simulink model "ACC_TEST_AEB_TEST_2011"  (Simulink 7.7)
settings: Solver=ode1  SolverMode=SingleTasking  StartTime=0.0  StopTime=T  FixedStep=0.001  RelTol=1e-3
PostLoadFcn:
  | , if any(exist('dsrtsu_mdlpostloadfcn', 'file') == [2, 3, 6]), try dsrtsu_mdlpostloadfcn('Execute', bdroot); catch fprintf('Error in PostLoadFcn (dsrtsu_mdlpostloadfcn) for model "%s":\n %s\n', bdroot, lasterr); end, end,
model workspace (MATLAB code in the model file):
  | % Define the sample time, |Ts|, and simulation duration, |T|, in seconds.
  | Ts = 0.1;
  | T = 35;
  | 
  | % Specify the initial position and velocity for the two vehicles.
  | % v0_lead_long = 20;
  | v0_lead_long = 15;
  | v0_lead_lat = 1;  % initial velocity for lead car (m/s)
  | x0_target = 45.15;            % Initial x position of target car          (m)
  | y0_target = 1.933;       % Initial y position of target car          (m)
  | % x0_target = 0;            % Initial x position of target car          (m)
  | % y0_target = 0;       % Initial y position of target car          (m)
  | lead_heading = 0.09;
  | yaw_des = 0.09;
  | 
  | % Initial condition for the ego car
  | x0_egoVehicle = [0 0];   % initial position for ego car (m)
  | v0_ego = 20;   % initial velocity for ego car (m/s)
  | % Initial condition for the ego car
  | % v0_ego = 20.6;         % Initial speed of the ego car           (m/s)
  | x0_ego = 0;            % Initial x position of ego car          (m)
  | y0_ego = 0;       % Initial y position of ego car          (m)
  | 
  | t_gap = 1.4;
  | D_default = 10;
  | %%
  | % Specify the driver-set velocity in m/s.
  | % v_set = 30;
  | 
  | %%
  | % Considering the physical limitations of the vehicle dynamics, the
  | % acceleration is constrained to the range  |[-3,2]| (m/s^2).
  | min_ac = -3;
  | max_ac = 2;
  | max_jerk = 90;
  | min_jerk =-90;
  | R           = 500;      % Radius of curvature for the road      (m)
  | %% Ego Car
  | % Dynamics modeling parameters
  | m       = 1575;     % Total mass of vehicle                          (kg)
  | Iz      = 2875;     % Yaw moment of inertia of vehicle               (m*N*s^2)
  | lf      = 1.2;      % Longitudinal distance from c.g. to front tires (m)
  | lr      = 1.6;      % Longitudinal distance from c.g. to rear tires  (m)
  | Cf      = 19000;    % Cornering stiffness of front tires             (N/rad)
  | Cr      = 33000;    % Cornering stiffness of rear tires              (N/rad)
  | tau     = 0.5;      % Longitudinal time constant                     (N/A)
  | 
  | % System matrices
  | A = [-(2*Cf+2*Cr)/m/v0_ego,0,-v0_ego-(2*Cf*lf-2*Cr*lr)/m/v0_ego,0,0;...
  |      0,0,1,0,0;...
  |      -(2*Cf*lf-2*Cr*lr)/Iz/v0_ego,0,-(2*Cf*lf^2+2*Cr*lr^2)/Iz/v0_ego,0,0;...
  |      0,0,0,0,1;...
  |      0,0,0,0,-1/tau];
  | % B1 = [2*Cf/m,0,2*Cf*lf/Iz,0,0]';
  | B2 = [0,0,0,0,1/tau]';
  | 
  | %% Linear Model for ACC design
  | % Input:  u (required longitudinal acceleration)
  | % Output: x4(longitudinal velocity)
  | C = [0,0,0,1,0];
  | G = minreal(ss(A,B2,C,0));
  | 
  | %% Driver steering control paramaters
  | driver_P        = 0.2;  % Proportional gain                     (N/A)
  | driver_I        = 0.1;  % Integral gain                         (N/A)
  | yawerr_gain     = 2;    % Yaw error gain                        (N/A)
  | 
  | %% Automatic Cruise Control (ACC) Controller Parameters
  | v_set           = 20; % ACC set speed                         (m/s)
  | time_gap        = 1;  % ACC time gap                          (s)
  | default_spacing = 5;    % ACC default spacing                   (m)
  | verr_gain       = 5;  % ACC velocity error gain               (N/A)
  | xerr_gain       = 0.2;  % ACC spacing error gain                (N/A)
  | vx_gain         = 0.1;  % ACC relative velocity gain            (N/A)
  | 
  | %% AEB
  | tau1     = 0.5;     % Longitudinal time constant (throttle)          (N/A)
  | tau2     = 0.07;    % Longitudinal time constant (brake)             (N/A)
  | v_set_aeb = 20;
  | 
  | %% Speed Controller Parameters
  | speedController.Kp = 1.1;           % Proportional Gain of speed controller
  | speedController.Ki = 0.1;           % Integral Gain of speed controller
  | speedController.Amax = 3;           % Maximum acceleration                  (m/s^2)
  | speedController.Amin = -3;          % Minimum acceleration                  (m/s^2)
  | 
  | %% FCW parameters
  | FCW.timeToReact  = 1.2;         % driver reaction time                   (sec)
  | FCW.driver_decel = 4.0;         % driver braking deceleration            (m/s^2)
  | 
  | %% AEB controller parameters
  | AEB.PB1_decel = 3.8;            % 1st stage Partial Braking deceleration (m/s^2)
  | AEB.PB2_decel = 5.3;            % 2nd stage Partial Braking deceleration (m/s^2)
  | AEB.FB_decel  = 9.8;            % Full Braking deceleration              (m/s^2)
  | AEB.headwayOffset = 3.7;        % headway offset                         (m)
  | AEB.timeMargin = 0;             % headway time margin                    (sec)
libraries: simulink x4
Description:
  | Standard RTI1401 template.
  | Supported Matlab version:  R2017a.
settings Model: Tag=RTI1401  DSRTSU_INTERNAL_RTI_VER=510  DSRTSU_INTERNAL_RTI_TYPE=rti1401  RTICANMMDATA=struct('GeneralSetupData',struct('modelroot',['C:\Users\pegas\Desktop\MDS\Desktop\Matlab Ex'],'generalsettings',struct('filesettings',struct('destfolder',struct('Name','RTICANMM_FILES','Check',1),'buildfolder',struct('Name','.','Check',1),'AbsDestfolder',struct('Name',['C:\Users\pegas\Desktop\MDS\Desktop\Matlab Ex\RTICANMM_FILES']),'AbsBuildfolder',struct('Name',['C:\Users\pegas\Desktop\MDS\Desktop\Matlab Ex']))),'options',struct('addpaths',1,'rmpaths',1,'addtrcexclusion',logical(1),'cannavigator',struct('checkmonitoring',0),'show_usrtrc',0,'use_usrtrc',0),'advanced',struct('options',[1 1 1 1 1 1 1 1 1 1 1 1 1 1 1 1 1 1 1 1 1 1 1 1 1 1 1 1 1 1 1 1 1 1 1 1 1 1 1 1 1 1 1 1 1 1 1 1 1 1 1 1 1 1 1 1 1 1 1 1 1 1 1 1 1 1 1 1 1 1 1 1 1 1 1 1 1 1 1 1 1 1 1 1 1 1 1 1 1 1 1 1 1 1 1 1 1 1 1 1]),'MPSetup',{{}},'modelname','ACC_TEST_AEB_TEST_2017','block','ACC_TEST_AEB_TEST_2017'))  DSRTSU_INTERNAL_RTIFLEXRAYCONFIG=110  DSRTSU_INTERNAL_RTIFPGA=110  Creator=pegas  LastModifiedBy=pegas  CovMetricSettings=dswe  CovHtmlReporting=off  covSaveCumulativeToWorkspaceVar=off  CovSaveSingleToWorkspaceVar=off  CovExternalEMLEnable=on
settings DataIOCC: LimitDataPoints=off  SaveFormat=StructureWithTime  SignalLoggingSaveFormat=Dataset
settings OptimizationCC: BlockReduction=off  OptimizeBlockIOStorage=off  BufferReuse=off  ExpressionFolding=off  ExpressionDepthLimit=128  LocalBlockOutputs=off
settings DebuggingCC: UnderspecifiedInitializationDetection=Simplified  MergeDetectMultiDrivingBlocksExec=error  SolverPrmCheckMsg=none  FcnCallInpInsideContextMsg=Enable All  StateNameClashWarn=none  SFUnexpectedBacktrackingDiag=error  SFNoUnconditionalDefaultTransitionDiag=error
settings HardwareCC: ProdLargestAtomicInteger=Integer  ProdLargestAtomicFloat=Float  ProdIntDivRoundTo=Zero  ProdEndianess=BigEndian  ProdHWDeviceType=Custom Processor->Custom  TargetIntDivRoundTo=Zero  TargetEndianess=BigEndian  TargetHWDeviceType=Custom Processor->Custom
settings RTWCC: SystemTargetFile=rti1401.tlc  MakeCommand=make_rti  TemplateMakefile=rti1401.tmf  Description=dSPACE DS1401 Hardware Platform
settings CodeAppCC: CustomSymbolStrType=$N$R$M_T
settings STFCustomTargetCC: TargetFunctionLibrary=C89/C90 (ANSI)  ParMdlRefBuildCompliant=on  MatFileLogging=on  SystemTargetFile=rti1401.tlc
settings GRTTargetCC: TargetFunctionLibrary=C89/C90 (ANSI)  CompOptLevelCompliant=off  GeneratePreprocessorConditionals=Use local settings
settings CustomProperty: DataType=RTWOptions_EnumType_C__Program Files_dSPACE RCPHIL 2017-B_MATLAB_RTI_RTI1401_TLC_rti1401_1InitialSimState  Value=RUN
settings EnumStrPairs: String=RUN

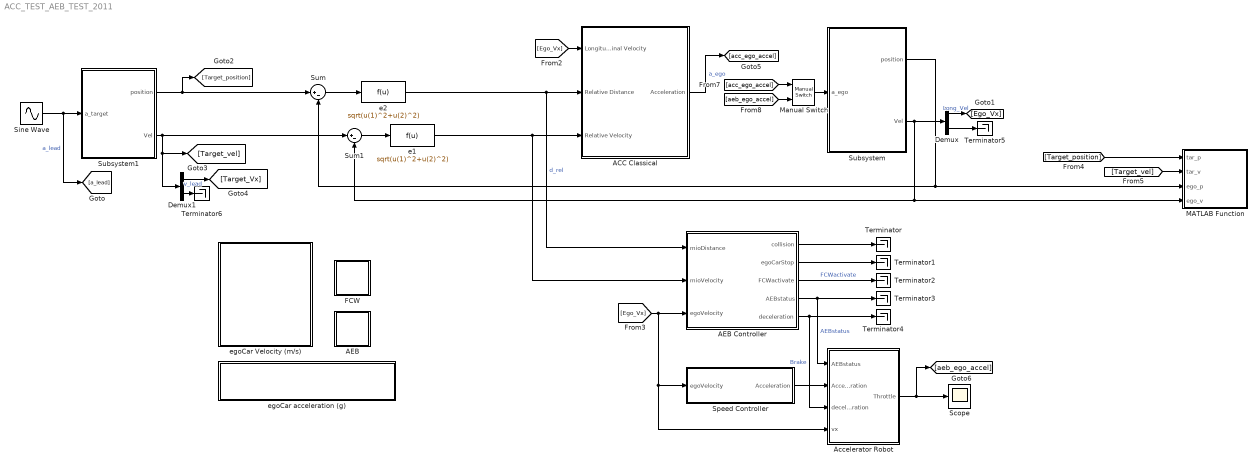
== system ACC_TEST_AEB_TEST_2011 ==
  ACC Classical : Subsystem  TreatAsAtomicUnit=on  VariantObject=controller_type == 1
      settings: RTWFileNameOpts=Use function name
  AEB : Subsystem  Description=Replaced Block
      mask Type: Replaced Block
      mask Description: This block has been replaced with an empty subsystem because it used functionality that is unavailable in Simulink R2011a.
      mask Display: fprintf('Replaced: %s\n','Dashboard Widget')
  AEB Controller : Subsystem
  Accelerator Robot : Subsystem
  Demux : Demux  Outputs=2
  Demux1 : Demux  Outputs=2
  FCW : Subsystem  Description=Replaced Block
      mask Type: Replaced Block
      mask Description: This block has been replaced with an empty subsystem because it used functionality that is unavailable in Simulink R2011a.
      mask Display: fprintf('Replaced: %s\n','Dashboard Widget')
  MATLAB Function : Stateflow chart  TreatAsAtomicUnit=on
      settings: PermitHierarchicalResolution=ParametersOnly
  Manual Switch : simulink/Signal Routing/Manual Switch  sw=1  action=0  varsize=off
  Scope : Scope
      settings: TimeRange=auto  MaxDataPoints=5000  SaveToWorkspace=off  YMin=-1.25  YMax=1.25  SampleTime=-1
  Sine Wave : Sin  Amplitude=0.6  Frequency=0.2  SampleTime=Ts
  Speed Controller : Subsystem
  Subsystem : Subsystem
  Subsystem1 : Subsystem
  Sum : Sum  Inputs=|+-
  Sum1 : Sum  Inputs=|+-
  Terminator{,1..6} (7 alike) : Terminator
  e1 : Fcn  Expr=sqrt(u(1)^2+u(2)^2)
  e2 : Fcn  Expr=sqrt(u(1)^2+u(2)^2)
  egoCar Velocity (m/s) : Subsystem  Description=Replaced Block
      mask Type: Replaced Block
      mask Description: This block has been replaced with an empty subsystem because it used functionality that is unavailable in Simulink R2011a.
      mask Display: fprintf('Replaced: %s\n','Dashboard Widget')
  egoCar acceleration (g) : Subsystem  Description=Replaced Block
      mask Type: Replaced Block
      mask Description: This block has been replaced with an empty subsystem because it used functionality that is unavailable in Simulink R2011a.
      mask Display: fprintf('Replaced: %s\n','Dashboard Widget')
  wires:
  Sum1/1 -> e1/1
  Sum/1 -> e2/1
  Subsystem1/1(position) -> [Target_position], Sum/1
  Subsystem1/2(Vel) -> Sum1/1, [Target_vel], Demux1/1
  Subsystem/2(Vel) -> Sum1/2, MATLAB Function/4(ego_v), Demux/1
  e1/1 -> ACC Classical/3(Relative Velocity), AEB Controller/2(mioVelocity)
  Subsystem/1(position) -> Sum/2, MATLAB Function/3(ego_p)
  Sine Wave/1 -> [a_lead], Subsystem1/1(a_target)  "a_lead"
  e2/1 -> ACC Classical/2(Relative Distance), AEB Controller/1(mioDistance)  "d_rel"
  AEB Controller/1(collision) -> Terminator/1
  AEB Controller/2(egoCarStop) -> Terminator1/1
  AEB Controller/3(FCWactivate) -> Terminator2/1  "FCWactivate"
  AEB Controller/4(AEBstatus) -> Terminator3/1, Accelerator Robot/1(AEBstatus)  "AEBstatus"
  AEB Controller/5(deceleration) -> Terminator4/1, Accelerator Robot/3(decelleration)  "Brake"
  Demux/2 -> Terminator5/1
  Demux/1 -> [Ego_Vx]  "Long_Vel"
  Speed Controller/1(Acceleration) -> Accelerator Robot/2(Acceleration)
  Accelerator Robot/1(Throttle) -> [aeb_ego_accel], Scope/1
  ACC Classical/1(Acceleration) -> [acc_ego_accel]  "a_ego"
  [Ego_Vx] -> ACC Classical/1(Longitudinal Velocity)
  [Ego_Vx] -> AEB Controller/3(egoVelocity), Accelerator Robot/4(vx), Speed Controller/1(egoVelocity)
  [Target_position] -> MATLAB Function/1(tar_p)
  [Target_vel] -> MATLAB Function/2(tar_v)
  Demux1/2 -> Terminator6/1
  Demux1/1 -> [Target_Vx]  "v_lead"
  Manual Switch/1 -> Subsystem/1(a_ego)
  [acc_ego_accel] -> Manual Switch/1
  [aeb_ego_accel] -> Manual Switch/2

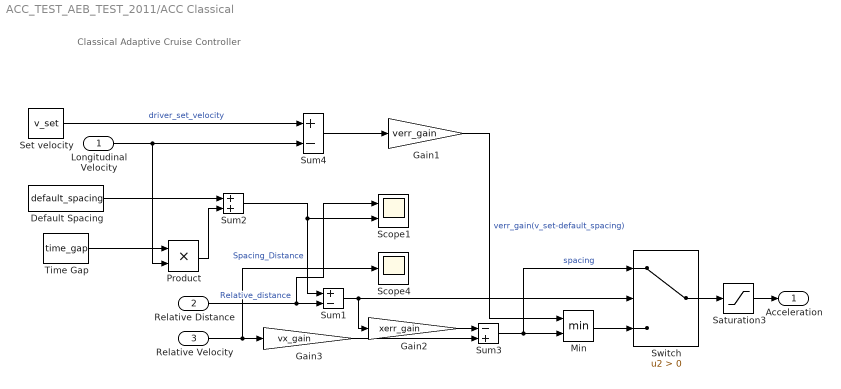
== system ACC_TEST_AEB_TEST_2011/ACC Classical ==
  note: Classical Adaptive Cruise Controller
  Longitudinal Velocity : Inport
  Relative Distance : Inport  Port=2
  Relative Velocity : Inport  Port=3
  Default Spacing : Constant  Value=default_spacing  SampleTime=Ts
  Gain1 : Gain  Gain=verr_gain
  Gain2 : Gain  Gain=xerr_gain
  Gain3 : Gain  Gain=vx_gain
  Min : MinMax  Inputs=2
  Product : Product
  Saturation3 : Saturate  UpperLimit=max_ac  LowerLimit=min_ac
  Scope1 : Scope  NumInputPorts=2
      settings: TimeRange=auto  MaxDataPoints=5000  SaveToWorkspace=off  YMin=-3.97675~-5  YMax=50.65448~5  SampleTime=-1
  Scope4 : Scope
      settings: TimeRange=auto  MaxDataPoints=5000  SaveToWorkspace=off  SaveName=ScopeData6  YMin=-0.54934  YMax=6.34874  SampleTime=-1
  Set velocity : Constant  Value=v_set  SampleTime=Ts
  Sum1 : Sum  Inputs=+-
  Sum2 : Sum
  Sum3 : Sum  Inputs=-+
  Sum4 : Sum  Inputs=+-
  Switch : Switch  Criteria=u2 > Threshold
  Time Gap : Constant  Value=time_gap  SampleTime=Ts
  Acceleration : Outport
  wires:
  Longitudinal Velocity/1 -> Product/2, Sum4/2
  Default Spacing/1 -> Sum2/1
  Gain2/1 -> Sum3/1
  Sum4/1 -> Gain1/1
  Gain3/1 -> Sum3/2
  Relative Velocity/1 -> Scope4/1, Gain3/1
  Time Gap/1 -> Product/1
  Switch/1 -> Saturation3/1
  Product/1 -> Sum2/2
  Set velocity/1 -> Sum4/1  "driver_set_velocity"
  Sum3/1 -> Switch/1, Min/2  "spacing"
  Sum1/1 -> Gain2/1, Switch/2
  Gain1/1 -> Min/1  "verr_gain(v_set-default_spacing)"
  Relative Distance/1 -> Scope1/1, Sum1/2  "Relative_distance"
  Sum2/1 -> Scope1/2, Sum1/1  "Spacing_Distance"
  Saturation3/1 -> Acceleration/1
  Min/1 -> Switch/3

== system ACC_TEST_AEB_TEST_2011/AEB ==

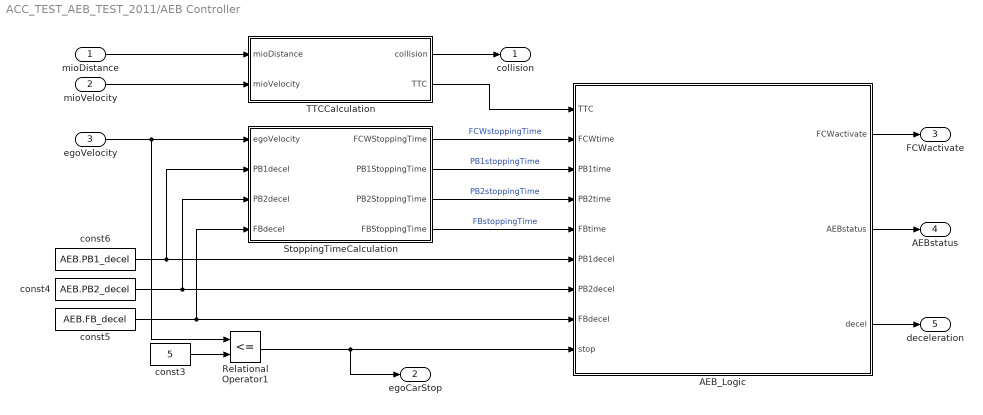
== system ACC_TEST_AEB_TEST_2011/AEB Controller ==
  mioDistance : Inport
  mioVelocity : Inport  Port=2
  egoVelocity : Inport  Port=3
  AEB_Logic : Stateflow chart  TreatAsAtomicUnit=on
      settings: PermitHierarchicalResolution=ParametersOnly
  Relational Operator1 : RelationalOperator  Operator=<=  OutDataTypeStr=boolean
  StoppingTimeCalculation : Subsystem
  TTCCalculation : Subsystem
  const3 : Constant  Value=5  SampleTime=-1
  const4 : Constant  Value=AEB.PB2_decel  SampleTime=-1
  const5 : Constant  Value=AEB.FB_decel  SampleTime=-1
  const6 : Constant  Value=AEB.PB1_decel  SampleTime=-1
  collision : Outport
  egoCarStop : Outport  Port=2
  FCWactivate : Outport  Port=3
  AEBstatus : Outport  Port=4
  deceleration : Outport  Port=5
  wires:
  AEB_Logic/3(decel) -> deceleration/1
  egoVelocity/1 -> StoppingTimeCalculation/1(egoVelocity), Relational Operator1/1
  const4/1 -> AEB_Logic/7(PB2decel), StoppingTimeCalculation/3(PB2decel)
  const5/1 -> StoppingTimeCalculation/4(FBdecel), AEB_Logic/8(FBdecel)
  AEB_Logic/2(AEBstatus) -> AEBstatus/1
  const3/1 -> Relational Operator1/2
  Relational Operator1/1 -> egoCarStop/1, AEB_Logic/9(stop)
  const6/1 -> AEB_Logic/6(PB1decel), StoppingTimeCalculation/2(PB1decel)
  StoppingTimeCalculation/3(PB2StoppingTime) -> AEB_Logic/4(PB2time)  "PB2stoppingTime"
  StoppingTimeCalculation/2(PB1StoppingTime) -> AEB_Logic/3(PB1time)  "PB1stoppingTime"
  StoppingTimeCalculation/4(FBStoppingTime) -> AEB_Logic/5(FBtime)  "FBstoppingTime"
  StoppingTimeCalculation/1(FCWStoppingTime) -> AEB_Logic/2(FCWtime)  "FCWstoppingTime"
  AEB_Logic/1(FCWactivate) -> FCWactivate/1
  mioDistance/1 -> TTCCalculation/1(mioDistance)
  mioVelocity/1 -> TTCCalculation/2(mioVelocity)
  TTCCalculation/1(collision) -> collision/1
  TTCCalculation/2(TTC) -> AEB_Logic/1(TTC)

== system ACC_TEST_AEB_TEST_2011/Accelerator Robot ==
  note: Robot release accelerator when AEB is activated
  AEBstatus : Inport
  Acceleration : Inport  Port=2
  decelleration : Inport  Port=3
  vx : Inport  Port=4
  Constant : Constant  Value=0
  Saturation : Saturate  UpperLimit=1  LowerLimit=-1
  Simple Driveline & Brakes : Subsystem
  Switch : Switch  Criteria=u2 > Threshold
  Throttle : Outport
  wires:
  Constant/1 -> Switch/1
  decelleration/1 -> Simple Driveline & Brakes/2(Brake)
  Switch/1 -> Simple Driveline & Brakes/1(Throttle)
  Simple Driveline & Brakes/1(Accel) -> Saturation/1
  Acceleration/1 -> Switch/3
  vx/1 -> Simple Driveline & Brakes/3(xdot)
  Saturation/1 -> Throttle/1
  AEBstatus/1 -> Switch/2

== system ACC_TEST_AEB_TEST_2011/FCW ==

== system ACC_TEST_AEB_TEST_2011/Speed Controller ==
  egoVelocity : Inport
  Discrete PID Controller2 : simulink/Continuous/PID Controller  Controller=PI  TimeDomain=Discrete-time  SampleTime=-1  IntegratorMethod=Forward Euler  FilterMethod=Forward Euler  Form=Parallel  UseFilter=on  ControllerParametersSource=internal  P=speedController.Kp  I=speedController.Ki  D=speedController.Kd  N=speedController.FilterCoeff  InitialConditionSource=internal  InitialConditionForIntegrator=0  InitialConditionForFilter=0  ExternalReset=none  LimitOutput=on  UpperSaturationLimit=speedController.Amax  LowerSaturationLimit=speedController.Amin  LinearizeAsGain=off  AntiWindupMode=clamping  Kb=1  TrackingMode=off  Kt=1  PParamMin=[]  PParamMax=[]  IParamMin=[]  IParamMax=[]  DParamMin=[]  DParamMax=[]  NParamMin=[]  NParamMax=[]  KbParamMin=[]  KbParamMax=[]  KtParamMin=[]  KtParamMax=[]  POutMin=[]  POutMax=[]  IOutMin=[]  IOutMax=[]  DOutMin=[]  DOutMax=[]  NOutMin=[]  NOutMax=[]  KbOutMin=[]  KbOutMax=[]  KtOutMin=[]  KtOutMax=[]  IntegratorOutMin=[]  IntegratorOutMax=[]  FilterOutMin=[]  FilterOutMax=[]  SumOutMin=[]  SumOutMax=[]  SumI1OutMin=[]  SumI1OutMax=[]  SumI2OutMin=[]  SumI2OutMax=[]  SumI3OutMin=[]  SumI3OutMax=[]  SumDOutMin=[]  SumDOutMax=[]  SaturationOutMin=[]  SaturationOutMax=[]  IntegratorContinuousStateAttributes=''  IntegratorStateMustResolveToSignalObject=off  IntegratorRTWStateStorageClass=Auto  FilterContinuousStateAttributes=''  FilterStateMustResolveToSignalObject=off  FilterRTWStateStorageClass=Auto  DifferentiatorICPrevScaledInput=0  DifferentiatorOutMin=[]  DifferentiatorOutMax=[]
  Set velocity : Constant  Value=v_set_aeb  SampleTime=Ts
  Sum4 : Sum  Inputs=+-
  Acceleration : Outport
  wires:
  Set velocity/1 -> Sum4/1  "driver_set_velocity"
  egoVelocity/1 -> Sum4/2
  Discrete PID Controller2/1 -> Acceleration/1
  Sum4/1 -> Discrete PID Controller2/1

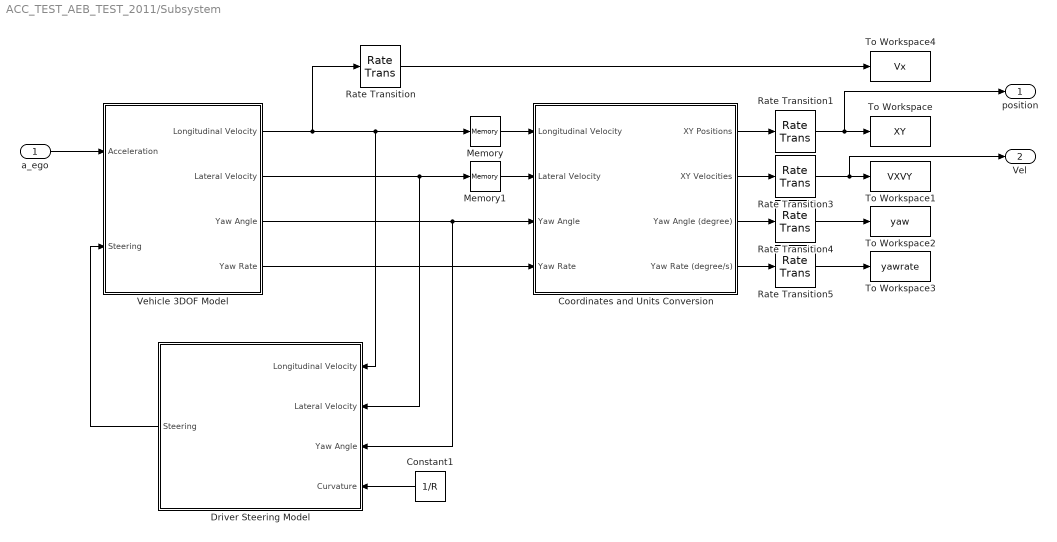
== system ACC_TEST_AEB_TEST_2011/Subsystem ==
  a_ego : Inport
  "  Vehicle 3DOF Model " : Subsystem
  Constant1 : Constant  Value=1/R
  Coordinates and Units Conversion : Subsystem
  Driver Steering Model : Subsystem
  Memory : Memory  X0=v0_ego
  Memory1 : Memory
  Rate Transition{,1,3..5} (5 alike) : RateTransition  OutPortSampleTime=Ts
  To Workspace : ToWorkspace  VariableName=XY  SaveFormat=Structure With Time  SampleTime=-1
  To Workspace1 : ToWorkspace  VariableName=VXVY  SaveFormat=Structure With Time  SampleTime=-1
  To Workspace2 : ToWorkspace  VariableName=yaw  SaveFormat=Structure With Time  SampleTime=-1
  To Workspace3 : ToWorkspace  VariableName=yawrate  SaveFormat=Structure With Time  SampleTime=-1
  To Workspace4 : ToWorkspace  VariableName=Vx  SaveFormat=Structure With Time  SampleTime=-1
  position : Outport
  Vel : Outport  Port=2
  wires:
  Coordinates and Units Conversion/3(Yaw Angle (degree)) -> Rate Transition4/1
  Rate Transition5/1 -> To Workspace3/1
  "  Vehicle 3DOF Model "/2(Lateral Velocity) -> Memory1/1, Driver Steering Model/2(Lateral Velocity)
  Rate Transition/1 -> To Workspace4/1
  Constant1/1 -> Driver Steering Model/4(Curvature)
  Coordinates and Units Conversion/1(XY Positions) -> Rate Transition1/1
  "  Vehicle 3DOF Model "/1(Longitudinal Velocity) -> Rate Transition/1, Driver Steering Model/1(Longitudinal Velocity), Memory/1
  Driver Steering Model/1(Steering) -> "  Vehicle 3DOF Model "/2(Steering)
  Rate Transition4/1 -> To Workspace2/1
  "  Vehicle 3DOF Model "/3(Yaw Angle) -> Coordinates and Units Conversion/3(Yaw Angle), Driver Steering Model/3(Yaw Angle)
  Coordinates and Units Conversion/4(Yaw Rate (degree/s)) -> Rate Transition5/1
  "  Vehicle 3DOF Model "/4(Yaw Rate) -> Coordinates and Units Conversion/4(Yaw Rate)
  Coordinates and Units Conversion/2(XY Velocities) -> Rate Transition3/1
  a_ego/1 -> "  Vehicle 3DOF Model "/1(Acceleration)
  Rate Transition1/1 -> position/1, To Workspace/1
  Rate Transition3/1 -> Vel/1, To Workspace1/1
  Memory/1 -> Coordinates and Units Conversion/1(Longitudinal Velocity)
  Memory1/1 -> Coordinates and Units Conversion/2(Lateral Velocity)

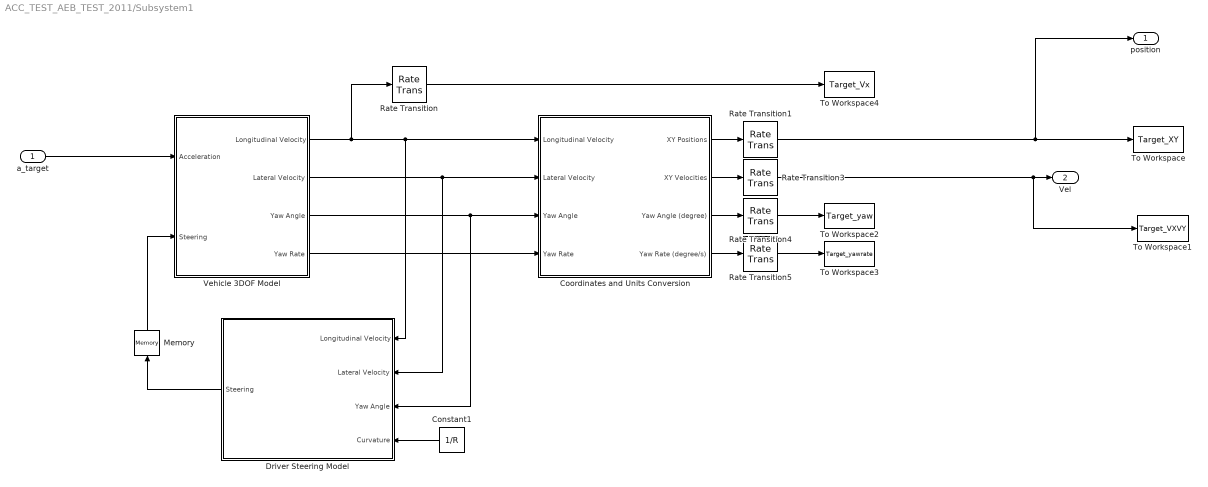
== system ACC_TEST_AEB_TEST_2011/Subsystem1 ==
  a_target : Inport
  "  Vehicle 3DOF Model " : Subsystem
  Constant1 : Constant  Value=1/R
  Coordinates and Units Conversion : Subsystem
  Driver Steering Model : Subsystem
  Memory : Memory  X0=0.01
  Rate Transition{,1,3..5} (5 alike) : RateTransition  OutPortSampleTime=Ts
  To Workspace : ToWorkspace  VariableName=Target_XY  SaveFormat=Structure With Time  SampleTime=-1
  To Workspace1 : ToWorkspace  VariableName=Target_VXVY  SaveFormat=Structure With Time  SampleTime=-1
  To Workspace2 : ToWorkspace  VariableName=Target_yaw  SaveFormat=Structure With Time  SampleTime=-1
  To Workspace3 : ToWorkspace  VariableName=Target_yawrate  SaveFormat=Structure With Time  SampleTime=-1
  To Workspace4 : ToWorkspace  VariableName=Target_Vx  SaveFormat=Structure With Time  SampleTime=-1
  position : Outport
  Vel : Outport  Port=2
  wires:
  a_target/1 -> "  Vehicle 3DOF Model "/1(Acceleration)
  Coordinates and Units Conversion/2(XY Velocities) -> Rate Transition3/1
  "  Vehicle 3DOF Model "/4(Yaw Rate) -> Coordinates and Units Conversion/4(Yaw Rate)
  Coordinates and Units Conversion/4(Yaw Rate (degree/s)) -> Rate Transition5/1
  "  Vehicle 3DOF Model "/3(Yaw Angle) -> Driver Steering Model/3(Yaw Angle), Coordinates and Units Conversion/3(Yaw Angle)
  Rate Transition4/1 -> To Workspace2/1
  Coordinates and Units Conversion/1(XY Positions) -> Rate Transition1/1
  Constant1/1 -> Driver Steering Model/4(Curvature)
  Rate Transition/1 -> To Workspace4/1
  Rate Transition5/1 -> To Workspace3/1
  Coordinates and Units Conversion/3(Yaw Angle (degree)) -> Rate Transition4/1
  Rate Transition1/1 -> position/1, To Workspace/1
  Rate Transition3/1 -> To Workspace1/1, Vel/1
  "  Vehicle 3DOF Model "/1(Longitudinal Velocity) -> Coordinates and Units Conversion/1(Longitudinal Velocity), Driver Steering Model/1(Longitudinal Velocity), Rate Transition/1
  "  Vehicle 3DOF Model "/2(Lateral Velocity) -> Coordinates and Units Conversion/2(Lateral Velocity), Driver Steering Model/2(Lateral Velocity)
  Driver Steering Model/1(Steering) -> Memory/1
  Memory/1 -> "  Vehicle 3DOF Model "/2(Steering)

== system ACC_TEST_AEB_TEST_2011/egoCar Velocity (m/s) ==

== system ACC_TEST_AEB_TEST_2011/egoCar acceleration (g) ==

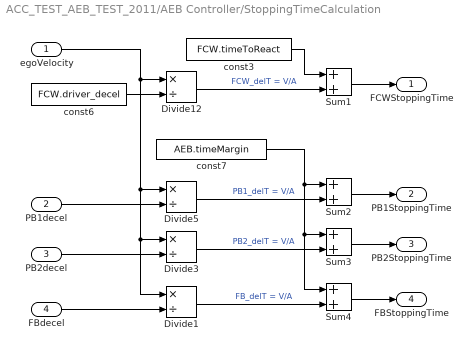
== system ACC_TEST_AEB_TEST_2011/AEB Controller/StoppingTimeCalculation ==
  egoVelocity : Inport
  PB1decel : Inport  Port=2
  PB2decel : Inport  Port=3
  FBdecel : Inport  Port=4
  Divide{1,3,5,12} (4 alike) : Product  Inputs=*/
  Sum{1..4} (4 alike) : Sum
  const3 : Constant  Value=FCW.timeToReact  SampleTime=-1
  const6 : Constant  Value=FCW.driver_decel  SampleTime=-1
  const7 : Constant  Value=AEB.timeMargin  SampleTime=-1
  FCWStoppingTime : Outport
  PB1StoppingTime : Outport  Port=2
  PB2StoppingTime : Outport  Port=3
  FBStoppingTime : Outport  Port=4
  wires:
  Sum1/1 -> FCWStoppingTime/1
  Sum2/1 -> PB1StoppingTime/1
  Sum3/1 -> PB2StoppingTime/1
  Sum4/1 -> FBStoppingTime/1
  const7/1 -> Sum2/1, Sum4/1, Sum3/1
  egoVelocity/1 -> Divide1/1, Divide3/1, Divide5/1, Divide12/1
  Divide5/1 -> Sum2/2  "PB1_delT = V/A"
  Divide3/1 -> Sum3/2  "PB2_delT = V/A"
  Divide1/1 -> Sum4/2  "FB_delT = V/A"
  const6/1 -> Divide12/2
  PB1decel/1 -> Divide5/2
  PB2decel/1 -> Divide3/2
  FBdecel/1 -> Divide1/2
  const3/1 -> Sum1/1
  Divide12/1 -> Sum1/2  "FCW_delT = V/A"

== system ACC_TEST_AEB_TEST_2011/AEB Controller/TTCCalculation ==
  mioDistance : Inport
  mioVelocity : Inport  Port=2
  Abs : Abs
  Divide11 : Product  Inputs=**
  Divide3 : Product  Inputs=*/
  Relational Operator : RelationalOperator  Operator=<  OutDataTypeStr=boolean
  Saturation : Saturate  UpperLimit=100  LowerLimit=0.01
  Sign : Signum
  Sum : Sum  Inputs=+-
  const1 : Constant  Value=AEB.headwayOffset  SampleTime=-1
  const2 : Constant  Value=0.1  SampleTime=-1
  collision : Outport
  TTC : Outport  Port=2
  wires:
  mioVelocity/1 -> Sign/1, Abs/1
  mioDistance/1 -> Sum/1
  Divide3/1 -> Divide11/1  "TTC"
  const1/1 -> Sum/2
  Sum/1 -> Relational Operator/1, Divide3/1  "headway"
  const2/1 -> Relational Operator/2
  Abs/1 -> Saturation/1
  Relational Operator/1 -> collision/1
  Saturation/1 -> Divide3/2
  Sign/1 -> Divide11/2
  Divide11/1 -> TTC/1  "TTC"

== system ACC_TEST_AEB_TEST_2011/Accelerator Robot/Simple Driveline & Brakes ==
  Throttle : Inport
  Brake : Inport  Port=2
  xdot : Inport  Port=3
  Gain : Gain  Gain=m
  Gain1 : Gain  Gain=0.8
  Gain2 : Gain  Gain=m
  Lower level dynamics1 : TransferFcn  Denominator=[tau1 1]
  Lower level dynamics2 : TransferFcn  Denominator=[tau2 1]
  Product : Product
  Subtract1 : Sum  Inputs=+-
  Trigonometric Function : Trigonometry  Operator=tanh
  Accel : Outport
  wires:
  Brake/1 -> Product/1
  Throttle/1 -> Gain/1
  Gain2/1 -> Lower level dynamics2/1
  Gain/1 -> Lower level dynamics1/1
  Subtract1/1 -> Accel/1
  xdot/1 -> Gain1/1
  Product/1 -> Gain2/1
  Trigonometric Function/1 -> Product/2
  Gain1/1 -> Trigonometric Function/1
  Lower level dynamics1/1 -> Subtract1/1
  Lower level dynamics2/1 -> Subtract1/2

== system ACC_TEST_AEB_TEST_2011/Subsystem/  Vehicle 3DOF Model  ==
  note: Vehicle 3DOF Model
  Acceleration : Inport
  Steering : Inport  Port=2
  Vehicle Dynamics : Subsystem
  Longitudinal Velocity : Outport
  Lateral Velocity : Outport  Port=2
  Yaw Angle : Outport  Port=3
  Yaw Rate : Outport  Port=4
  wires:
  Steering/1 -> Vehicle Dynamics/2(Steering)
  Acceleration/1 -> Vehicle Dynamics/1(Acceleration)
  Vehicle Dynamics/1(Longitudinal Velocity) -> Longitudinal Velocity/1
  Vehicle Dynamics/2(Lateral Velocity) -> Lateral Velocity/1
  Vehicle Dynamics/3(Yaw Angle) -> Yaw Angle/1
  Vehicle Dynamics/4(Yaw Rate) -> Yaw Rate/1

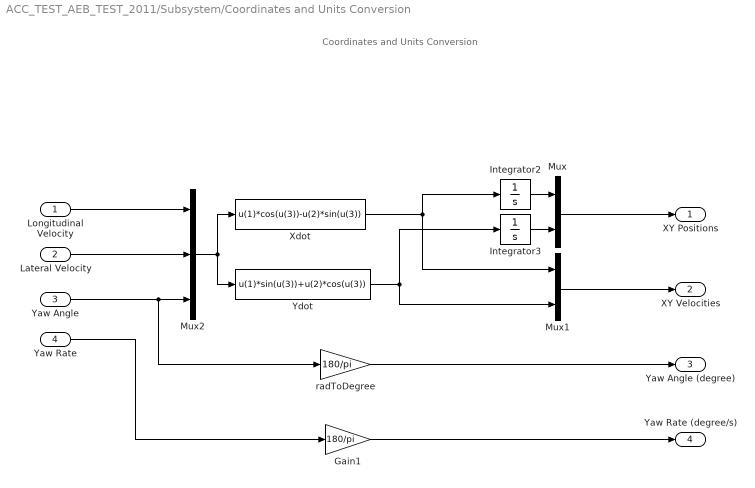
== system ACC_TEST_AEB_TEST_2011/Subsystem/Coordinates and Units Conversion ==
  note: Coordinates and Units Conversion
  Longitudinal Velocity : Inport
  Lateral Velocity : Inport  Port=2
  Yaw Angle : Inport  Port=3
  Yaw Rate : Inport  Port=4
  Gain1 : Gain  Gain=180/pi
  Integrator2 : Integrator  InitialCondition=x0_ego
  Integrator3 : Integrator  InitialCondition=y0_ego
  Mux : Mux  Inputs=2
  Mux1 : Mux  Inputs=2
  Mux2 : Mux  Inputs=3
  Xdot : Fcn  Expr=u(1)*cos(u(3))-u(2)*sin(u(3))
  Ydot : Fcn  Expr=u(1)*sin(u(3))+u(2)*cos(u(3))
  "radToDegree " : Gain  Gain=180/pi
  XY Positions : Outport
  XY Velocities : Outport  Port=2
  Yaw Angle (degree) : Outport  Port=3
  Yaw Rate (degree/s) : Outport  Port=4
  wires:
  "radToDegree "/1 -> Yaw Angle (degree)/1
  Integrator2/1 -> Mux/1
  Mux/1 -> XY Positions/1
  Ydot/1 -> Mux1/2, Integrator3/1
  Gain1/1 -> Yaw Rate (degree/s)/1
  Yaw Rate/1 -> Gain1/1
  Integrator3/1 -> Mux/2
  Xdot/1 -> Integrator2/1, Mux1/1
  Mux1/1 -> XY Velocities/1
  Lateral Velocity/1 -> Mux2/2
  Mux2/1 -> Ydot/1, Xdot/1
  Longitudinal Velocity/1 -> Mux2/1
  Yaw Angle/1 -> "radToDegree "/1, Mux2/3

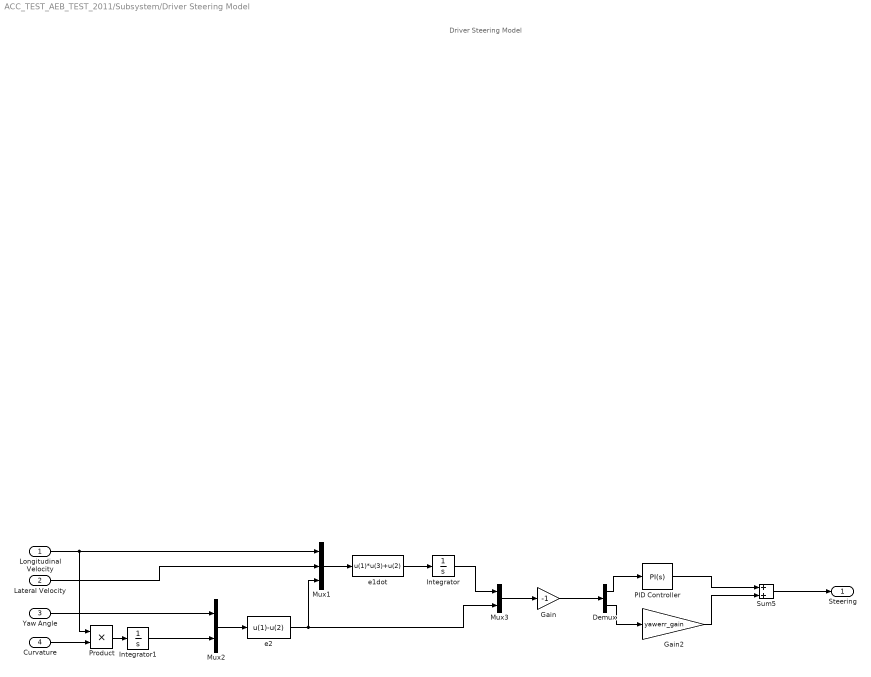
== system ACC_TEST_AEB_TEST_2011/Subsystem/Driver Steering Model ==
  note: Driver Steering Model
  Longitudinal Velocity : Inport
  Lateral Velocity : Inport  Port=2
  Yaw Angle : Inport  Port=3
  Curvature : Inport  Port=4
  Demux : Demux  Outputs=2
  Gain : Gain  Gain=-1
  Gain2 : Gain  Gain=yawerr_gain
  Integrator : Integrator
  Integrator1 : Integrator
  Mux1 : Mux  Inputs=3
  Mux2 : Mux  Inputs=2
  Mux3 : Mux  Inputs=2
  PID Controller : simulink/Continuous/PID Controller  Controller=PI  TimeDomain=Continuous-time  SampleTime=-1  IntegratorMethod=Forward Euler  FilterMethod=Forward Euler  Form=Parallel  UseFilter=on  ControllerParametersSource=internal  P=driver_P  I=driver_I  D=0  N=100  InitialConditionSource=internal  InitialConditionForIntegrator=0  InitialConditionForFilter=0  ExternalReset=none  LimitOutput=off  UpperSaturationLimit=inf  LowerSaturationLimit=-inf  LinearizeAsGain=on  AntiWindupMode=none  Kb=1  TrackingMode=off  Kt=1  PParamMin=[]  PParamMax=[]  IParamMin=[]  IParamMax=[]  DParamMin=[]  DParamMax=[]  NParamMin=[]  NParamMax=[]  KbParamMin=[]  KbParamMax=[]  KtParamMin=[]  KtParamMax=[]  POutMin=[]  POutMax=[]  IOutMin=[]  IOutMax=[]  DOutMin=[]  DOutMax=[]  NOutMin=[]  NOutMax=[]  KbOutMin=[]  KbOutMax=[]  KtOutMin=[]  KtOutMax=[]  IntegratorOutMin=[]  IntegratorOutMax=[]  FilterOutMin=[]  FilterOutMax=[]  SumOutMin=[]  SumOutMax=[]  SumI1OutMin=[]  SumI1OutMax=[]  SumI2OutMin=[]  SumI2OutMax=[]  SumI3OutMin=[]  SumI3OutMax=[]  SumDOutMin=[]  SumDOutMax=[]  SaturationOutMin=[]  SaturationOutMax=[]  IntegratorContinuousStateAttributes=''  IntegratorStateMustResolveToSignalObject=off  IntegratorRTWStateStorageClass=Auto  FilterContinuousStateAttributes=''  FilterStateMustResolveToSignalObject=off  FilterRTWStateStorageClass=Auto  DifferentiatorICPrevScaledInput=0  DifferentiatorOutMin=[]  DifferentiatorOutMax=[]
  Product : Product
  Sum5 : Sum
  e1dot : Fcn  Expr=u(1)*u(3)+u(2)
  e2 : Fcn  Expr=u(1)-u(2)
  Steering : Outport
  wires:
  e1dot/1 -> Integrator/1
  Mux2/1 -> e2/1
  e2/1 -> Mux1/3, Mux3/2
  Mux3/1 -> Gain/1
  Lateral Velocity/1 -> Mux1/2
  Yaw Angle/1 -> Mux2/1
  Mux1/1 -> e1dot/1
  Integrator/1 -> Mux3/1
  Product/1 -> Integrator1/1
  Integrator1/1 -> Mux2/2
  Curvature/1 -> Product/2
  Longitudinal Velocity/1 -> Product/1, Mux1/1
  Gain2/1 -> Sum5/2
  PID Controller/1 -> Sum5/1
  Demux/2 -> Gain2/1
  Sum5/1 -> Steering/1
  Demux/1 -> PID Controller/1
  Gain/1 -> Demux/1

== system ACC_TEST_AEB_TEST_2011/Subsystem1/  Vehicle 3DOF Model  ==
  note: Vehicle 3DOF Model
  Acceleration : Inport
  Steering : Inport  Port=2
  Vehicle Dynamics : Subsystem
  Longitudinal Velocity : Outport
  Lateral Velocity : Outport  Port=2
  Yaw Angle : Outport  Port=3
  Yaw Rate : Outport  Port=4
  wires:
  Vehicle Dynamics/4(Yaw Rate) -> Yaw Rate/1
  Vehicle Dynamics/3(Yaw Angle) -> Yaw Angle/1
  Vehicle Dynamics/2(Lateral Velocity) -> Lateral Velocity/1
  Vehicle Dynamics/1(Longitudinal Velocity) -> Longitudinal Velocity/1
  Acceleration/1 -> Vehicle Dynamics/1(Acceleration)
  Steering/1 -> Vehicle Dynamics/2(Steering)

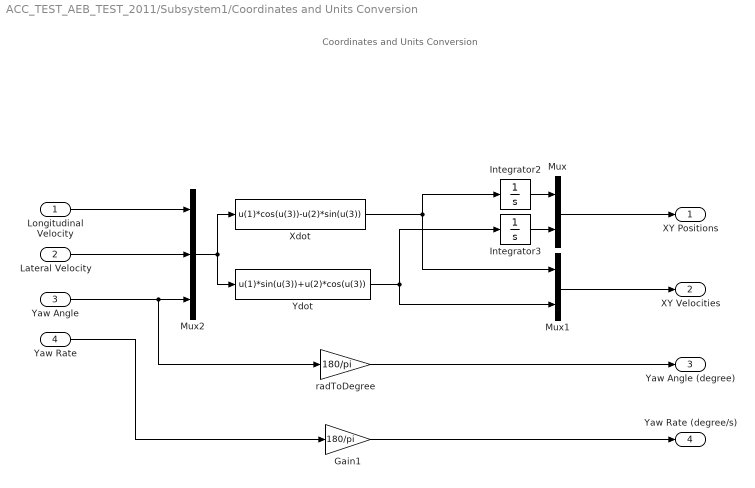
== system ACC_TEST_AEB_TEST_2011/Subsystem1/Coordinates and Units Conversion ==
  note: Coordinates and Units Conversion
  Longitudinal Velocity : Inport
  Lateral Velocity : Inport  Port=2
  Yaw Angle : Inport  Port=3
  Yaw Rate : Inport  Port=4
  Gain1 : Gain  Gain=180/pi
  Integrator2 : Integrator  InitialCondition=x0_target
  Integrator3 : Integrator  InitialCondition=y0_target
  Mux : Mux  Inputs=2
  Mux1 : Mux  Inputs=2
  Mux2 : Mux  Inputs=3
  Xdot : Fcn  Expr=u(1)*cos(u(3))-u(2)*sin(u(3))
  Ydot : Fcn  Expr=u(1)*sin(u(3))+u(2)*cos(u(3))
  "radToDegree " : Gain  Gain=180/pi
  XY Positions : Outport
  XY Velocities : Outport  Port=2
  Yaw Angle (degree) : Outport  Port=3
  Yaw Rate (degree/s) : Outport  Port=4
  wires:
  Yaw Angle/1 -> Mux2/3, "radToDegree "/1
  Longitudinal Velocity/1 -> Mux2/1
  Mux2/1 -> Xdot/1, Ydot/1
  Lateral Velocity/1 -> Mux2/2
  Mux1/1 -> XY Velocities/1
  Xdot/1 -> Mux1/1, Integrator2/1
  Integrator3/1 -> Mux/2
  Yaw Rate/1 -> Gain1/1
  Gain1/1 -> Yaw Rate (degree/s)/1
  Ydot/1 -> Integrator3/1, Mux1/2
  Mux/1 -> XY Positions/1
  Integrator2/1 -> Mux/1
  "radToDegree "/1 -> Yaw Angle (degree)/1

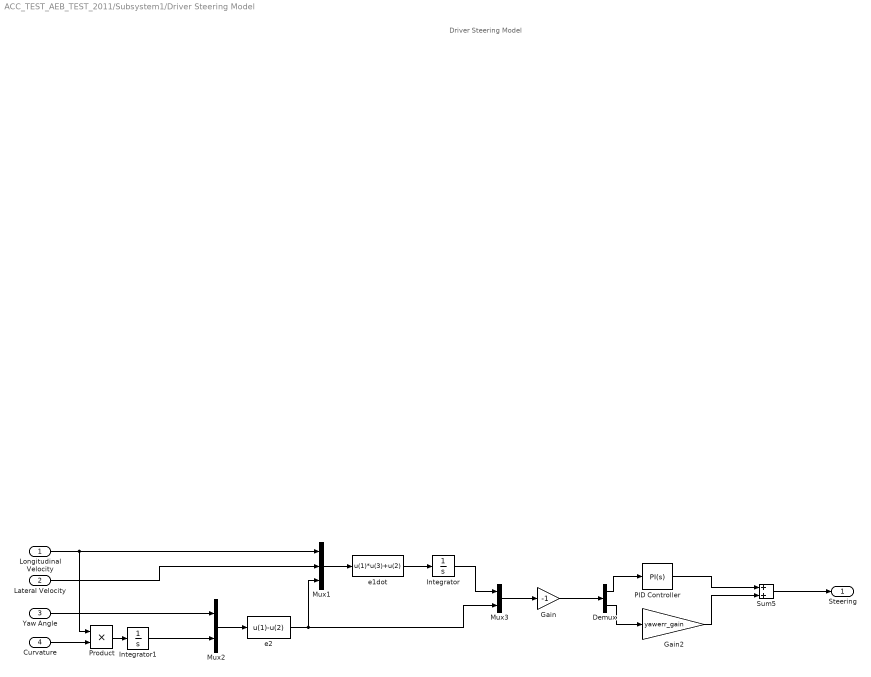
== system ACC_TEST_AEB_TEST_2011/Subsystem1/Driver Steering Model ==
  note: Driver Steering Model
  Longitudinal Velocity : Inport
  Lateral Velocity : Inport  Port=2
  Yaw Angle : Inport  Port=3
  Curvature : Inport  Port=4
  Demux : Demux  Outputs=2
  Gain : Gain  Gain=-1
  Gain2 : Gain  Gain=yawerr_gain
  Integrator : Integrator
  Integrator1 : Integrator  InitialCondition=yaw_des
  Mux1 : Mux  Inputs=3
  Mux2 : Mux  Inputs=2
  Mux3 : Mux  Inputs=2
  PID Controller : simulink/Continuous/PID Controller  Controller=PI  TimeDomain=Continuous-time  SampleTime=-1  IntegratorMethod=Forward Euler  FilterMethod=Forward Euler  Form=Parallel  UseFilter=on  ControllerParametersSource=internal  P=driver_P  I=driver_I  D=0  N=100  InitialConditionSource=internal  InitialConditionForIntegrator=0  InitialConditionForFilter=0  ExternalReset=none  LimitOutput=off  UpperSaturationLimit=inf  LowerSaturationLimit=-inf  LinearizeAsGain=on  AntiWindupMode=none  Kb=1  TrackingMode=off  Kt=1  PParamMin=[]  PParamMax=[]  IParamMin=[]  IParamMax=[]  DParamMin=[]  DParamMax=[]  NParamMin=[]  NParamMax=[]  KbParamMin=[]  KbParamMax=[]  KtParamMin=[]  KtParamMax=[]  POutMin=[]  POutMax=[]  IOutMin=[]  IOutMax=[]  DOutMin=[]  DOutMax=[]  NOutMin=[]  NOutMax=[]  KbOutMin=[]  KbOutMax=[]  KtOutMin=[]  KtOutMax=[]  IntegratorOutMin=[]  IntegratorOutMax=[]  FilterOutMin=[]  FilterOutMax=[]  SumOutMin=[]  SumOutMax=[]  SumI1OutMin=[]  SumI1OutMax=[]  SumI2OutMin=[]  SumI2OutMax=[]  SumI3OutMin=[]  SumI3OutMax=[]  SumDOutMin=[]  SumDOutMax=[]  SaturationOutMin=[]  SaturationOutMax=[]  IntegratorContinuousStateAttributes=''  IntegratorStateMustResolveToSignalObject=off  IntegratorRTWStateStorageClass=Auto  FilterContinuousStateAttributes=''  FilterStateMustResolveToSignalObject=off  FilterRTWStateStorageClass=Auto  DifferentiatorICPrevScaledInput=0  DifferentiatorOutMin=[]  DifferentiatorOutMax=[]
  Product : Product
  Sum5 : Sum
  e1dot : Fcn  Expr=u(1)*u(3)+u(2)
  e2 : Fcn  Expr=u(1)-u(2)
  Steering : Outport
  wires:
  Gain/1 -> Demux/1
  Demux/1 -> PID Controller/1
  Demux/2 -> Gain2/1
  PID Controller/1 -> Sum5/1
  Gain2/1 -> Sum5/2
  Longitudinal Velocity/1 -> Mux1/1, Product/1
  Curvature/1 -> Product/2
  Integrator1/1 -> Mux2/2
  Product/1 -> Integrator1/1
  Integrator/1 -> Mux3/1
  Mux1/1 -> e1dot/1
  Yaw Angle/1 -> Mux2/1
  Lateral Velocity/1 -> Mux1/2
  Mux3/1 -> Gain/1
  e2/1 -> Mux3/2, Mux1/3
  Mux2/1 -> e2/1
  e1dot/1 -> Integrator/1
  Sum5/1 -> Steering/1

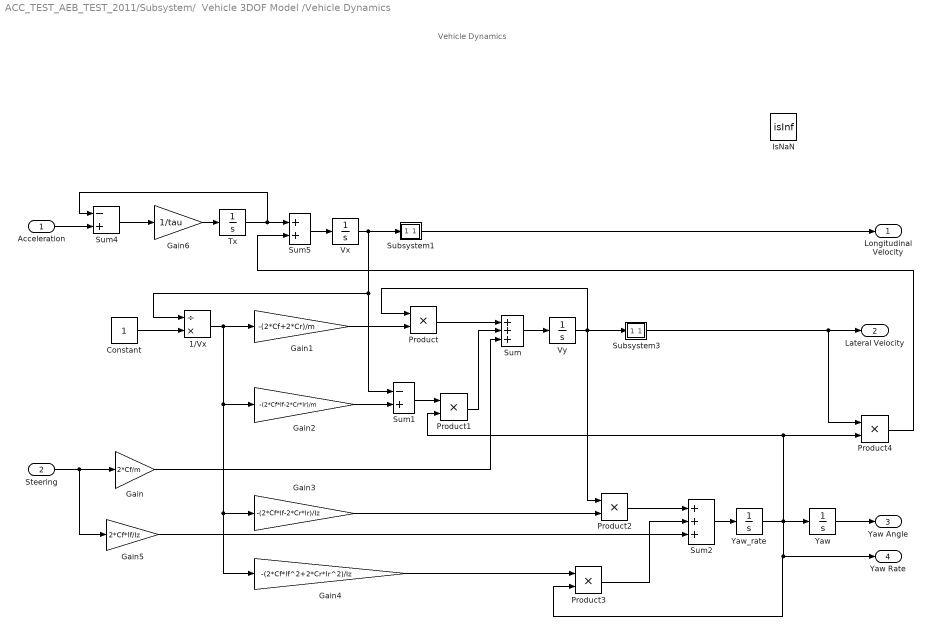
== system ACC_TEST_AEB_TEST_2011/Subsystem/  Vehicle 3DOF Model /Vehicle Dynamics ==
  note: Vehicle Dynamics
  Acceleration : Inport
  Steering : Inport  Port=2
  1/Vx : Product  Inputs=/*
  Constant : Constant
  Gain : Gain  Gain=2*Cf/m
  Gain1 : Gain  Gain=-(2*Cf+2*Cr)/m
  Gain2 : Gain  Gain=-(2*Cf*lf-2*Cr*lr)/m
  Gain3 : Gain  Gain=-(2*Cf*lf-2*Cr*lr)/Iz
  Gain4 : Gain  Gain=-(2*Cf*lf^2+2*Cr*lr^2)/Iz
  Gain5 : Gain  Gain=2*Cf*lf/Iz
  Gain6 : Gain  Gain=1/tau
  IsNaN : RelationalOperator  Operator=isInf  OutDataTypeStr=boolean
  Product{,1..4} (5 alike) : Product
  Subsystem1 : Subsystem
  Subsystem3 : Subsystem
  Sum : Sum  Inputs=+++
  Sum1 : Sum  Inputs=-+
  Sum2 : Sum  Inputs=+++
  Sum4 : Sum  Inputs=-+
  Sum5 : Sum
  Tx : Integrator
  Vx : Integrator  InitialCondition=v0_ego
  Vy : Integrator  InitialCondition=1
  Yaw : Integrator
  "Yaw_rate " : Integrator
  Longitudinal Velocity : Outport
  Lateral Velocity : Outport  Port=2
  Yaw Angle : Outport  Port=3
  Yaw Rate : Outport  Port=4
  wires:
  Gain6/1 -> Tx/1
  Sum2/1 -> "Yaw_rate "/1
  Sum5/1 -> Vx/1
  Gain2/1 -> Sum1/2
  Gain4/1 -> Product3/1
  Constant/1 -> 1/Vx/2
  Gain3/1 -> Product2/2
  1/Vx/1 -> Gain4/1, Gain3/1, Gain2/1, Gain1/1
  Product2/1 -> Sum2/1
  Sum4/1 -> Gain6/1
  Acceleration/1 -> Sum4/2
  Tx/1 -> Sum5/1, Sum4/1
  Product3/1 -> Sum2/2
  Gain5/1 -> Sum2/3
  Product4/1 -> Sum5/2
  Sum1/1 -> Product1/1
  "Yaw_rate "/1 -> Yaw Rate/1, Product3/2, Product4/2, Product1/2, Yaw/1
  Gain/1 -> Sum/3
  Yaw/1 -> Yaw Angle/1
  Steering/1 -> Gain/1, Gain5/1
  Gain1/1 -> Product/2
  Product/1 -> Sum/1
  Vy/1 -> Product/1, Subsystem3/1(In1), Product2/1
  Sum/1 -> Vy/1
  Vx/1 -> Subsystem1/1(In1), 1/Vx/1, Sum1/1
  Product1/1 -> Sum/2
  Subsystem3/1(Out1) -> Lateral Velocity/1, Product4/1
  Subsystem1/1(Out1) -> Longitudinal Velocity/1

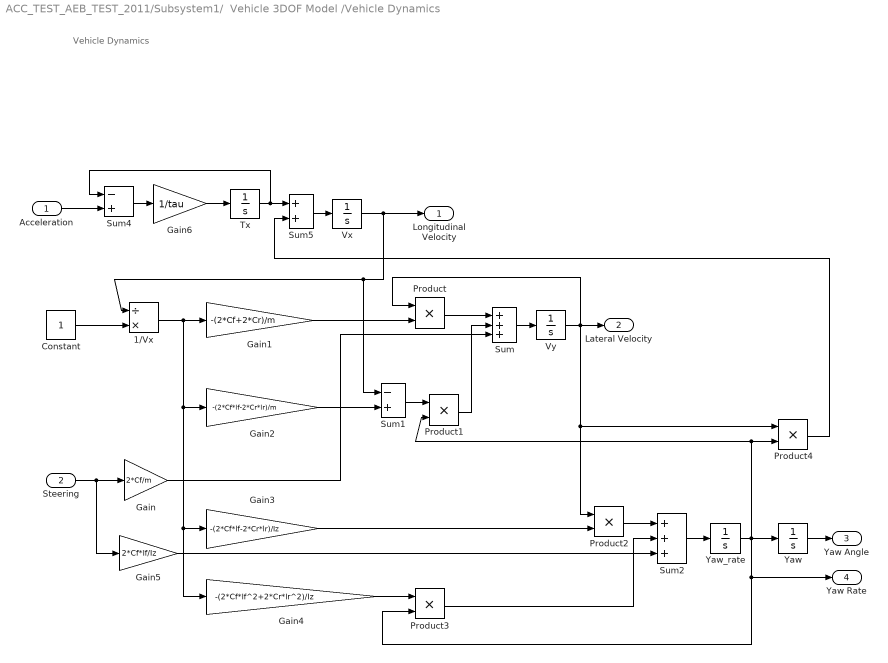
== system ACC_TEST_AEB_TEST_2011/Subsystem1/  Vehicle 3DOF Model /Vehicle Dynamics ==
  note: Vehicle Dynamics
  Acceleration : Inport
  Steering : Inport  Port=2
  1/Vx : Product  Inputs=/*
  Constant : Constant
  Gain : Gain  Gain=2*Cf/m
  Gain1 : Gain  Gain=-(2*Cf+2*Cr)/m
  Gain2 : Gain  Gain=-(2*Cf*lf-2*Cr*lr)/m
  Gain3 : Gain  Gain=-(2*Cf*lf-2*Cr*lr)/Iz
  Gain4 : Gain  Gain=-(2*Cf*lf^2+2*Cr*lr^2)/Iz
  Gain5 : Gain  Gain=2*Cf*lf/Iz
  Gain6 : Gain  Gain=1/tau
  Product{,1..4} (5 alike) : Product
  Sum : Sum  Inputs=+++
  Sum1 : Sum  Inputs=-+
  Sum2 : Sum  Inputs=+++
  Sum4 : Sum  Inputs=-+
  Sum5 : Sum
  Tx : Integrator
  Vx : Integrator  InitialCondition=v0_lead_long
  Vy : Integrator  InitialCondition=v0_lead_lat
  Yaw : Integrator  InitialCondition=lead_heading
  "Yaw_rate " : Integrator
  Longitudinal Velocity : Outport
  Lateral Velocity : Outport  Port=2
  Yaw Angle : Outport  Port=3
  Yaw Rate : Outport  Port=4
  wires:
  Product1/1 -> Sum/2
  Vx/1 -> Longitudinal Velocity/1, Sum1/1, 1/Vx/1
  Sum/1 -> Vy/1
  Vy/1 -> Product2/1, Product4/1, Lateral Velocity/1, Product/1
  Product/1 -> Sum/1
  Gain1/1 -> Product/2
  Steering/1 -> Gain5/1, Gain/1
  Yaw/1 -> Yaw Angle/1
  Gain/1 -> Sum/3
  "Yaw_rate "/1 -> Yaw/1, Yaw Rate/1, Product3/2, Product1/2, Product4/2
  Sum1/1 -> Product1/1
  Product4/1 -> Sum5/2
  Gain5/1 -> Sum2/3
  Product3/1 -> Sum2/2
  Tx/1 -> Sum5/1, Sum4/1
  Acceleration/1 -> Sum4/2
  Sum4/1 -> Gain6/1
  Product2/1 -> Sum2/1
  1/Vx/1 -> Gain1/1, Gain2/1, Gain3/1, Gain4/1
  Gain3/1 -> Product2/2
  Constant/1 -> 1/Vx/2
  Gain4/1 -> Product3/1
  Gain2/1 -> Sum1/2
  Sum5/1 -> Vx/1
  Sum2/1 -> "Yaw_rate "/1
  Gain6/1 -> Tx/1

== system ACC_TEST_AEB_TEST_2011/Subsystem/  Vehicle 3DOF Model /Vehicle Dynamics/Subsystem1 ==
  In1 : Inport
  If : If
  If Action Subsystem : Subsystem  TreatAsAtomicUnit=on
  If Action Subsystem1 : Subsystem  TreatAsAtomicUnit=on
  Merge : Merge
  Out1 : Outport
  wires:
  In1/1 -> If/1, If Action Subsystem1/1(In1), If Action Subsystem/1(In1)
  If Action Subsystem1/1(Out1) -> Merge/2
  If Action Subsystem/1(Out1) -> Merge/1
  If/2 -> If Action Subsystem1/Action
  If/1 -> If Action Subsystem/Action
  Merge/1 -> Out1/1

== system ACC_TEST_AEB_TEST_2011/Subsystem/  Vehicle 3DOF Model /Vehicle Dynamics/Subsystem3 ==
  In1 : Inport
  If : If
  If Action Subsystem : Subsystem  TreatAsAtomicUnit=on
  If Action Subsystem1 : Subsystem  TreatAsAtomicUnit=on
  Merge : Merge
  Out1 : Outport
  wires:
  Merge/1 -> Out1/1
  If/1 -> If Action Subsystem/Action
  If/2 -> If Action Subsystem1/Action
  If Action Subsystem/1(Out1) -> Merge/1
  If Action Subsystem1/1(Out1) -> Merge/2
  In1/1 -> If Action Subsystem/1(In1), If Action Subsystem1/1(In1), If/1

== system ACC_TEST_AEB_TEST_2011/Subsystem/  Vehicle 3DOF Model /Vehicle Dynamics/Subsystem1/If Action Subsystem ==
  In1 : Inport
  Action Port : ActionPort  ActionType=then
  Constant : Constant  Value=0.000000001
  Switch : Switch  Criteria=u2 > Threshold  Threshold=0.0001
  Out1 : Outport
  wires:
  Constant/1 -> Switch/3
  Switch/1 -> Out1/1
  In1/1 -> Switch/2, Switch/1

== system ACC_TEST_AEB_TEST_2011/Subsystem/  Vehicle 3DOF Model /Vehicle Dynamics/Subsystem1/If Action Subsystem1 ==
  In1 : Inport
  Action Port : ActionPort  ActionType=else
  Constant : Constant  Value=0.000000001
  Switch : Switch  Criteria=u2 > Threshold  Threshold=-0.0001
  Out1 : Outport
  wires:
  Switch/1 -> Out1/1
  Constant/1 -> Switch/1
  In1/1 -> Switch/2, Switch/3

== system ACC_TEST_AEB_TEST_2011/Subsystem/  Vehicle 3DOF Model /Vehicle Dynamics/Subsystem3/If Action Subsystem ==
  In1 : Inport
  Action Port : ActionPort  ActionType=then
  Constant : Constant  Value=0.000000001
  Switch : Switch  Criteria=u2 > Threshold  Threshold=0.0001
  Out1 : Outport
  wires:
  In1/1 -> Switch/1, Switch/2
  Switch/1 -> Out1/1
  Constant/1 -> Switch/3

== system ACC_TEST_AEB_TEST_2011/Subsystem/  Vehicle 3DOF Model /Vehicle Dynamics/Subsystem3/If Action Subsystem1 ==
  In1 : Inport
  Action Port : ActionPort  ActionType=else
  Constant : Constant  Value=0.000000001
  Switch : Switch  Criteria=u2 > Threshold  Threshold=-0.0001
  Out1 : Outport
  wires:
  In1/1 -> Switch/3, Switch/2
  Constant/1 -> Switch/1
  Switch/1 -> Out1/1

== matlab function MATLAB Function ==
  data: tar_p input double; tar_v input double; ego_p input double; ego_v input double
function fcn(tar_p,tar_v,ego_p,ego_v)
figure(1)
plot(tar_p(1),tar_p(2),'r.')
hold on
plot(ego_p(1),ego_p(2),'b.')
axis([0 550 0 550])


title('ACC/AEB Test')

% figure(1)
% plot(tar_p(1),tar_p(2),'.')
% hold on
% plot(ego_p(1),ego_p(2),'.')

== stateflow chart AEB Controller/AEB_Logic ==
  note: FCW/AEB Logic
  state Default
    entry: AEBstatus = 0;
    FCWactivate = 0;
    decel = 0;
  state FCW
    entry: AEBstatus = 0;
    FCWactivate = 1;
    decel = 0;
  state Partial_Braking1
    entry: AEBstatus = 1;
    FCWactivate = 1;
    decel = PB1decel;
  state Full_Braking
    entry: AEBstatus = 3;
    FCWactivate = 1;
    decel = FBdecel;
  state Partial_Braking2
    entry: AEBstatus = 2;
    FCWactivate = 1;
    decel = PB2decel;
  (default) -> Default
  Full_Braking -> Default [order 1] : [stop==1]
  Partial_Braking2 -> Default [order 2] : [stop==1]
  Partial_Braking1 -> Default [order 2] : [stop==1]
  Default -> FCW : [(abs(TTC)<FCWtime) ]
  FCW -> Default [order 2] : [abs(TTC)>=1.2*FCWtime]
  FCW -> Partial_Braking1 [order 1] : [(abs(TTC) < PB1time)]
  Partial_Braking1 -> FCW [order 3] : [abs(TTC)>=1.2*PB1time]
  Partial_Braking1 -> Partial_Braking2 [order 1] : [(abs(TTC) < PB2time) ]
  Partial_Braking2 -> Partial_Braking1 [order 3] : [abs(TTC)>=1.2*PB2time]
  Full_Braking -> Partial_Braking2 [order 2] : [abs(TTC)>=1.2*FBtime]
  Partial_Braking2 -> Full_Braking [order 1] : [(abs(TTC) < FBtime)]
  data: FCWactivate output double; TTC input double; FCWtime input double; PB1time input double; PB2time input double; FBtime input double; PB1decel input double; PB2decel input double; FBdecel input double; AEBstatus output double; decel output double; stop input double
